simulink model "zweipunktreglertest"  (R2016a)
settings: Solver=FixedStepAuto  StartTime=0.0  StopTime=800  RelTol=1e-3
settings Model: Creator=Hello Cao  LastModifiedBy=HaloCao
settings DataIOCC: LimitDataPoints=on  SaveFormat=Array
settings DebuggingCC: MaxConsecutiveZCsMsg=none
settings HardwareCC: ProdLargestAtomicFloat=None  ProdIntDivRoundTo=Undefined  ProdEndianess=Unspecified  ProdWordSize=32  ProdHWDeviceType=Generic->64-bit Embedded Processor (LLP64)  TargetBitPerPointer=64  TargetLongLongMode=on  TargetIntDivRoundTo=Zero  TargetEndianess=LittleEndian  TargetWordSize=64  TargetHWDeviceType=MATLAB Host  ProdEqTarget=off
settings ModelReferenceCC: PropagateSignalLabelsOutOfModel=off
settings ConfigComp: CovModelRefEnable=Off  CovSFcnEnable=off

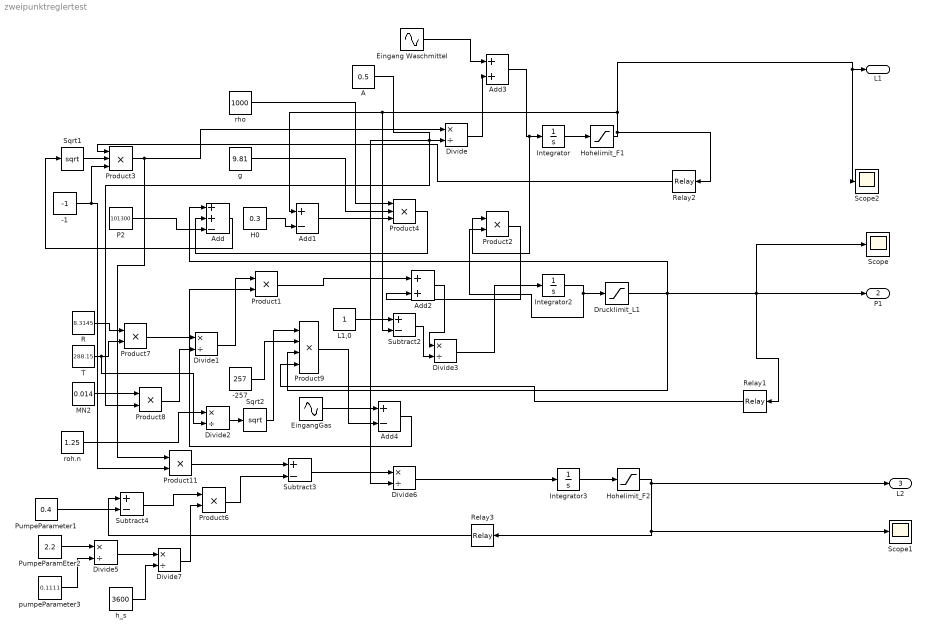
== system zweipunktreglertest ==
  -1 : Constant  Value=-1
  -257 : Constant  Value=257
  A : Constant  Value=0.5
  Add : Sum  Inputs=++-
  Add1 : Sum  Inputs=+-
  Add2 : Sum
  Add3 : Sum
  Add4 : Sum  Inputs=+-
  Divide{,1..3,5..7} (7 alike) : Product  Inputs=*/
  Drucklimit_L1 : Saturate  UpperLimit=3039000  LowerLimit=0
  Eingang Waschmittel : Sin  Amplitude=0.0001  Bias=0.001  SampleTime=0
  EingangGas : Sin  Amplitude=0.01  Bias=0.01  SampleTime=0
  H0 : Constant  Value=0.3
  Hohelimit_F1 : Saturate  UpperLimit=0.9  LowerLimit=0
  Hohelimit_F2 : Saturate  UpperLimit=0.9  LowerLimit=0
  Integrator : Integrator
  Integrator2 : Integrator  InitialCondition=3000000
  Integrator3 : Integrator
  L1,0 : Constant
  MN2 : Constant  Value=0.014
  P2 : Constant  Value=101300
  Product{1..2,6..8,11} (6 alike) : Product
  Product3 : Product  Inputs=3
  Product4 : Product  Inputs=3
  Product9 : Product  Inputs=4
  PumpeParamEter2 : Constant  Value=2.2
  PumpeParameter1 : Constant  Value=0.4
  R : Constant  Value=8.3145
  Relay1 : Relay  OnSwitchValue=709100  OffSwitchValue=690000  OnOutputValue=0.000000005
  Relay2 : Relay  OnSwitchValue=0.502  OffSwitchValue=0.499  OnOutputValue=0.000001
  Relay3 : Relay  OnSwitchValue=0.203  OffSwitchValue=0.193  OnOutputValue=0.8
  Scope : Scope
  Scope1 : Scope
  Scope2 : Scope
  Sqrt1 : Sqrt  SaturateOnIntegerOverflow=on
  Sqrt2 : Sqrt  SaturateOnIntegerOverflow=on
  Subtract2 : Sum  Inputs=+-
  Subtract3 : Sum  Inputs=+-
  Subtract4 : Sum  Inputs=+-
  T : Constant  Value=288.15
  g : Constant  Value=9.81
  h_s : Constant  Value=3600
  pumpeParameter3 : Constant  Value=0.1111
  rho : Constant  Value=1000
  roh.n : Constant  Value=1.25
  L1 : Outport
  P1 : Outport  Port=2
  L2 : Outport  Port=3
  wires:
  Integrator/1 -> Hohelimit_F1/1
  Sqrt1/1 -> Product3/2
  Add/1 -> Sqrt1/1
  H0/1 -> Add1/2
  rho/1 -> Product4/1
  g/1 -> Product4/2
  Add1/1 -> Product4/3
  Product4/1 -> Add/2
  P2/1 -> Add/3
  A/1 -> Divide6/2, Product8/2, Divide/2
  Divide/1 -> Add3/2
  R/1 -> Product7/1
  T/1 -> Divide2/2, Product7/2
  Product7/1 -> Divide1/1
  MN2/1 -> Product8/1
  Product8/1 -> Divide1/2
  -257/1 -> Product9/2
  Divide2/1 -> Sqrt2/1
  Sqrt2/1 -> Product9/1
  L1,0/1 -> Subtract2/1
  Subtract2/1 -> Divide3/2
  Divide3/1 -> Integrator2/1
  -1/1 -> Product11/2, Product3/3
  Product3/1 -> Product11/1, Divide/1
  Product11/1 -> Subtract3/1
  Product6/1 -> Subtract3/2
  Subtract4/1 -> Product6/1
  PumpeParameter1/1 -> Subtract4/2
  PumpeParamEter2/1 -> Divide5/1
  pumpeParameter3/1 -> Divide5/2
  Subtract3/1 -> Divide6/1
  Divide6/1 -> Integrator3/1
  Integrator2/1 -> Product2/2, Drucklimit_L1/1
  Integrator3/1 -> Hohelimit_F2/1
  Eingang Waschmittel/1 -> Add3/1
  Add3/1 -> Product2/1, Integrator/1
  EingangGas/1 -> Add4/1
  roh.n/1 -> Divide2/1
  Add4/1 -> Product1/2
  Divide1/1 -> Product1/1
  Divide5/1 -> Divide7/1
  Divide7/1 -> Product6/2
  h_s/1 -> Divide7/2
  Drucklimit_L1/1 -> Product9/3, Add/1, Relay1/1, Scope/1, P1/1
  Hohelimit_F1/1 -> Scope2/1, L1/1, Subtract2/2, Add1/1, Relay2/1
  Hohelimit_F2/1 -> Relay3/1, Scope1/1, L2/1
  Product9/1 -> Add4/2
  Relay1/1 -> Product9/4
  Relay2/1 -> Product3/1
  Relay3/1 -> Subtract4/1
  Product1/1 -> Add2/1
  Product2/1 -> Add2/2
  Add2/1 -> Divide3/1
